simulink model "DC_Motor_CoastMode_WithGearbox"  (R2019b)
settings: Solver=VariableStepAuto  StartTime=0.0  StopTime=10.0  FixedStep=1e-5  RelTol=1e-3
settings Model: Creator=Thomas  LastModifiedBy=thomas.jespersen
settings DataIOCC: ReturnWorkspaceOutputs=off
settings DebuggingCC: ArithmeticOperatorsInVariantConditions=warning
settings SFSimCC: SimUseLocalCustomCode=off  CustomCodeUndefinedFunction=UseInterfaceOnly
settings RTWCC: RTWUseLocalCustomCode=off

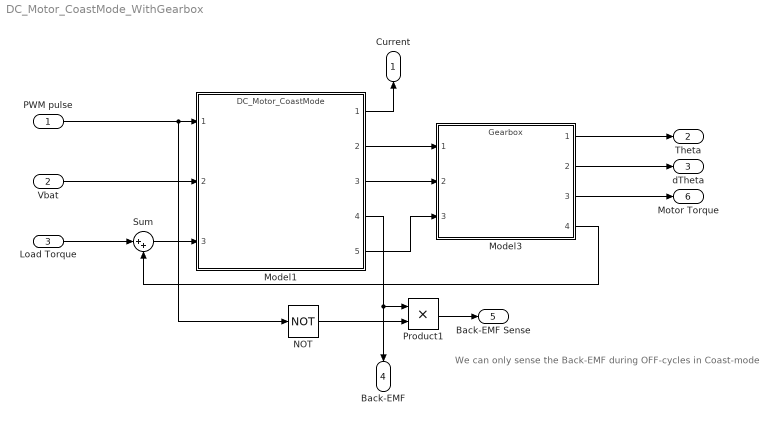
== system DC_Motor_CoastMode_WithGearbox ==
  note: We can only sense the Back-EMF during OFF-cycles in Coast-mode
  PWM pulse : Inport  OutDataTypeStr=int8
  Vbat : Inport  Port=2  OutDataTypeStr=double
  Load Torque : Inport  Port=3  OutDataTypeStr=double
  Model1 : ModelReference  ModelNameDialog=DC_Motor_CoastMode  SimulationMode=Normal  ModelReferenceVersion=1.43
  Model3 : ModelReference  ModelNameDialog=Gearbox  SimulationMode=Normal  ModelReferenceVersion=1.7
  NOT : Logic  Operator=NOT  IconShape=distinctive  AllPortsSameDT=off  OutDataTypeStr=boolean
  Product1 : Product
  Sum : Sum  Inputs=|++
  Current : Outport  VectorParamsAs1DForOutWhenUnconnected=off
  Theta : Outport  Port=2  VectorParamsAs1DForOutWhenUnconnected=off
  dTheta : Outport  Port=3  VectorParamsAs1DForOutWhenUnconnected=off
  Back-EMF : Outport  Port=4  VectorParamsAs1DForOutWhenUnconnected=off
  Back-EMF Sense : Outport  Port=5  VectorParamsAs1DForOutWhenUnconnected=off
  Motor Torque : Outport  Port=6  VectorParamsAs1DForOutWhenUnconnected=off
  wires:
  Vbat/1 -> Model1/2
  Model1/4 -> Back-EMF/1, Product1/1
  PWM pulse/1 -> NOT/1, Model1/1
  NOT/1 -> Product1/2
  Product1/1 -> Back-EMF Sense/1
  Model1/2 -> Model3/1
  Model1/3 -> Model3/2
  Model1/5 -> Model3/3
  Model1/1 -> Current/1
  Load Torque/1 -> Sum/1
  Sum/1 -> Model1/3
  Model3/4 -> Sum/2
  Model3/1 -> Theta/1
  Model3/2 -> dTheta/1
  Model3/3 -> Motor Torque/1
